simulink model "ER16_Simulation_Line_2020a"  (R2020a)
settings: Solver=ode15s  StartTime=0.0  StopTime=50  RelTol=1e-3
PreLoadFcn:
  | run('ER16_DataFile.m'); % 手动加载模型装配数据
model workspace: external: MATLAB File E:\Traj-tracking Simulation of ER16\Code\ER16_DataFile.m (data not in the file)
undefined symbols (not defined in the file): sigbuilder_block, smiData, X, Y, Z
libraries: sm_lib x49, nesl_utility x13
(part 2 of 2)

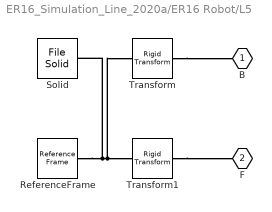
== system ER16_Simulation_Line_2020a/ER16 Robot/L5 ==
  ReferenceFrame : sm_lib/Frames and Transforms/Reference Frame
  Solid : sm_lib/Body Elements/File Solid  ExtGeomFileName=..\3D-Models\ER16_j5_默认_sldprt.STL  UnitType=Custom  ExtGeomFileUnits=mm  StepReaderType=HEX  ExportConvexHullGeometry=off  InertiaType=Custom  Mass=smiData.Solid(5).mass  MassUnits=kg  CenterOfMass=smiData.Solid(5).CoM  CenterOfMassUnits=mm  MomentsOfInertia=smiData.Solid(5).MoI  MomentsOfInertiaUnits=kg*mm^2  ProductsOfInertia=smiData.Solid(5).PoI  ProductsOfInertiaUnits=kg*mm^2  BasedOnType=DensityFromFile  Density=1000  DensityUnits=kg/m^3  DoExposeReferenceFrame=on  SerializedFrames=<Frames/>  GraphicType=FromGeometry  MarkerShape=Sphere  MarkerSize=10  GraphicVisPropType=SimpleVisualProperties  GraphicDiffuseColor=[0.82 0.49 0.11]  GraphicSpecularColor=[0.5 0.5 0.5 1.0]  GraphicAmbientColor=[0.15 0.15 0.15 1.0]  GraphicEmissiveColor=[0.0 0.0 0.0 1.0]  GraphicShininess=75  GraphicOpacity=smiData.Solid(5).opacity
  Transform : sm_lib/Frames and Transforms/Rigid Transform  TranslationMethod=Cartesian  TranslationStandardOffset=0  TranslationLengthUnit=mm  TranslationStandardAxis=+Z  TranslationCartesianOffset=smiData.RigidTransform(12).translation  TranslationROffset=0  TranslationROffsetUnits=m  TranslationZOffset=0  TranslationZOffsetUnits=m  TranslationThetaOffset=0  TranslationThetaOffsetUnits=deg  RotationMethod=ArbitraryAxis  RotationAngleUnits=rad  RotationStandardAxis=+Z  RotationAngle=smiData.RigidTransform(12).angle  RotationArbitraryAxis=smiData.RigidTransform(12).axis  FollAlignAxisA=+X  BaseAlignAxisA=+Y  FollAlignAxisB=+Y  BaseAlignAxisB=+Z  RotationSequenceAxes=FollowerAxes  RotationSequence=XYX  RotationSequenceAngles=[0 0 0]  RotationSequenceAnglesUnits=deg  RotationMatrix=[1 0 0; 0 1 0; 0 0 1]
  Transform1 : sm_lib/Frames and Transforms/Rigid Transform  TranslationMethod=Cartesian  TranslationStandardOffset=0  TranslationLengthUnit=mm  TranslationStandardAxis=+Z  TranslationCartesianOffset=smiData.RigidTransform(13).translation  TranslationROffset=0  TranslationROffsetUnits=m  TranslationZOffset=0  TranslationZOffsetUnits=m  TranslationThetaOffset=0  TranslationThetaOffsetUnits=deg  RotationMethod=ArbitraryAxis  RotationAngleUnits=rad  RotationStandardAxis=+Z  RotationAngle=smiData.RigidTransform(13).angle  RotationArbitraryAxis=smiData.RigidTransform(13).axis  FollAlignAxisA=+X  BaseAlignAxisA=+Y  FollAlignAxisB=+Y  BaseAlignAxisB=+Z  RotationSequenceAxes=FollowerAxes  RotationSequence=XYX  RotationSequenceAngles=[0 0 0]  RotationSequenceAnglesUnits=deg  RotationMatrix=[1 0 0; 0 1 0; 0 0 1]
  B : PMIOPort  Side=Left
  F : PMIOPort  Port=2  Side=Right
  connections:
  Solid/RConn1 -- ReferenceFrame/RConn1 -- Transform/LConn1 -- Transform1/LConn1
  Transform/RConn1 -- B/RConn1
  Transform1/RConn1 -- F/RConn1

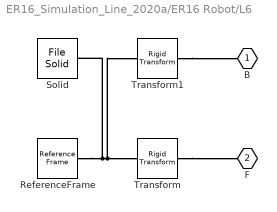
== system ER16_Simulation_Line_2020a/ER16 Robot/L6 ==
  ReferenceFrame : sm_lib/Frames and Transforms/Reference Frame
  Solid : sm_lib/Body Elements/File Solid  ExtGeomFileName=..\3D-Models\ER16_j6_默认_sldprt.STL  UnitType=Custom  ExtGeomFileUnits=mm  StepReaderType=HEX  ExportConvexHullGeometry=off  InertiaType=Custom  Mass=smiData.Solid(1).mass  MassUnits=kg  CenterOfMass=smiData.Solid(1).CoM  CenterOfMassUnits=mm  MomentsOfInertia=smiData.Solid(1).MoI  MomentsOfInertiaUnits=kg*mm^2  ProductsOfInertia=smiData.Solid(1).PoI  ProductsOfInertiaUnits=kg*mm^2  BasedOnType=DensityFromFile  Density=1000  DensityUnits=kg/m^3  DoExposeReferenceFrame=on  SerializedFrames=<Frames/>  GraphicType=FromGeometry  MarkerShape=Sphere  MarkerSize=10  GraphicVisPropType=SimpleVisualProperties  GraphicDiffuseColor=[0.82 0.49 0.11]  GraphicSpecularColor=[0.5 0.5 0.5 1.0]  GraphicAmbientColor=[0.15 0.15 0.15 1.0]  GraphicEmissiveColor=[0.0 0.0 0.0 1.0]  GraphicShininess=75  GraphicOpacity=smiData.Solid(1).opacity
  Transform : sm_lib/Frames and Transforms/Rigid Transform  TranslationMethod=Cartesian  TranslationStandardOffset=0  TranslationLengthUnit=mm  TranslationStandardAxis=+Z  TranslationCartesianOffset=smiData.RigidTransform(1).translation  TranslationROffset=0  TranslationROffsetUnits=m  TranslationZOffset=0  TranslationZOffsetUnits=m  TranslationThetaOffset=0  TranslationThetaOffsetUnits=deg  RotationMethod=ArbitraryAxis  RotationAngleUnits=rad  RotationStandardAxis=+Z  RotationAngle=smiData.RigidTransform(1).angle  RotationArbitraryAxis=smiData.RigidTransform(1).axis  FollAlignAxisA=+X  BaseAlignAxisA=+Y  FollAlignAxisB=+Y  BaseAlignAxisB=+Z  RotationSequenceAxes=FollowerAxes  RotationSequence=XYX  RotationSequenceAngles=[0 0 0]  RotationSequenceAnglesUnits=deg  RotationMatrix=[1 0 0; 0 1 0; 0 0 1]
  Transform1 : sm_lib/Frames and Transforms/Rigid Transform  TranslationMethod=Cartesian  TranslationStandardOffset=0  TranslationLengthUnit=mm  TranslationStandardAxis=+Z  TranslationCartesianOffset=smiData.RigidTransform(14).translation  TranslationROffset=0  TranslationROffsetUnits=m  TranslationZOffset=0  TranslationZOffsetUnits=m  TranslationThetaOffset=0  TranslationThetaOffsetUnits=deg  RotationMethod=ArbitraryAxis  RotationAngleUnits=rad  RotationStandardAxis=+Z  RotationAngle=smiData.RigidTransform(14).angle  RotationArbitraryAxis=smiData.RigidTransform(14).axis  FollAlignAxisA=+X  BaseAlignAxisA=+Y  FollAlignAxisB=+Y  BaseAlignAxisB=+Z  RotationSequenceAxes=FollowerAxes  RotationSequence=XYX  RotationSequenceAngles=[0 0 0]  RotationSequenceAnglesUnits=deg  RotationMatrix=[1 0 0; 0 1 0; 0 0 1]
  B : PMIOPort  Side=Left
  F : PMIOPort  Port=2  Side=Right
  connections:
  Solid/RConn1 -- ReferenceFrame/RConn1 -- Transform/LConn1 -- Transform1/LConn1
  Transform/RConn1 -- F/RConn1
  Transform1/RConn1 -- B/RConn1

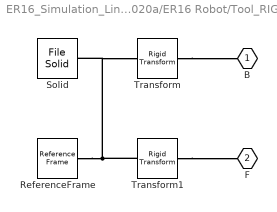
== system ER16_Simulation_Line_2020a/ER16 Robot/Tool_RIGID ==
  ReferenceFrame : sm_lib/Frames and Transforms/Reference Frame
  Solid : sm_lib/Body Elements/File Solid  ExtGeomFileName=..\3D-Models\Tool_默认_sldprt.STL  UnitType=Custom  ExtGeomFileUnits=mm  StepReaderType=HEX  ExportConvexHullGeometry=off  InertiaType=Custom  Mass=smiData.Solid(9).mass  MassUnits=kg  CenterOfMass=smiData.Solid(9).CoM  CenterOfMassUnits=mm  MomentsOfInertia=smiData.Solid(9).MoI  MomentsOfInertiaUnits=kg*mm^2  ProductsOfInertia=smiData.Solid(9).PoI  ProductsOfInertiaUnits=kg*mm^2  BasedOnType=DensityFromFile  Density=1000  DensityUnits=kg/m^3  DoExposeReferenceFrame=on  SerializedFrames=<Frames/>  GraphicType=FromGeometry  MarkerShape=Sphere  MarkerSize=10  GraphicVisPropType=SimpleVisualProperties  GraphicDiffuseColor=smiData.Solid(9).color  GraphicSpecularColor=[0.5 0.5 0.5 1.0]  GraphicAmbientColor=[0.15 0.15 0.15 1.0]  GraphicEmissiveColor=[0.0 0.0 0.0 1.0]  GraphicShininess=75  GraphicOpacity=smiData.Solid(9).opacity
  Transform : sm_lib/Frames and Transforms/Rigid Transform  TranslationMethod=Cartesian  TranslationStandardOffset=0  TranslationLengthUnit=mm  TranslationStandardAxis=+Z  TranslationCartesianOffset=smiData.RigidTransform(2).translation  TranslationROffset=0  TranslationROffsetUnits=m  TranslationZOffset=0  TranslationZOffsetUnits=m  TranslationThetaOffset=0  TranslationThetaOffsetUnits=deg  RotationMethod=ArbitraryAxis  RotationAngleUnits=rad  RotationStandardAxis=+Z  RotationAngle=smiData.RigidTransform(2).angle  RotationArbitraryAxis=smiData.RigidTransform(2).axis  FollAlignAxisA=+X  BaseAlignAxisA=+Y  FollAlignAxisB=+Y  BaseAlignAxisB=+Z  RotationSequenceAxes=FollowerAxes  RotationSequence=XYX  RotationSequenceAngles=[0 0 0]  RotationSequenceAnglesUnits=deg  RotationMatrix=[1 0 0; 0 1 0; 0 0 1]
  Transform1 : sm_lib/Frames and Transforms/Rigid Transform  TranslationMethod=Cartesian  TranslationStandardOffset=0.1325  TranslationLengthUnit=mm  TranslationStandardAxis=+X  TranslationCartesianOffset=smiData.RigidTransform(2).translation  TranslationROffset=0  TranslationROffsetUnits=m  TranslationZOffset=0  TranslationZOffsetUnits=m  TranslationThetaOffset=0  TranslationThetaOffsetUnits=deg  RotationMethod=ArbitraryAxis  RotationAngleUnits=rad  RotationStandardAxis=+Z  RotationAngle=0  RotationArbitraryAxis=smiData.RigidTransform(2).axis  FollAlignAxisA=+X  BaseAlignAxisA=+Y  FollAlignAxisB=+Y  BaseAlignAxisB=+Z  RotationSequenceAxes=FollowerAxes  RotationSequence=XYX  RotationSequenceAngles=[0 0 0]  RotationSequenceAnglesUnits=deg  RotationMatrix=[1 0 0; 0 1 0; 0 0 1]
  B : PMIOPort  Side=Left
  F : PMIOPort  Port=2  Side=Right
  connections:
  ReferenceFrame/RConn1 -- Transform1/LConn1 -- Transform/LConn1 -- Solid/RConn1
  Transform/RConn1 -- B/RConn1
  Transform1/RConn1 -- F/RConn1

== matlab function ER16_Simulation_Line_2020a/Calculator/Impedance Control Y ==
  settings: updateMethod=DISCRETE  sampleTime=0.005
  data: Y_Xd input; Y_Xr output; Y_Xr_d output; Y_Xr_dd output; Y_Xd_d input; Y_Xd_dd input; f input
function [Y_Xr,Y_Xr_d,Y_Xr_dd]  = fcnlmp(Y_Xd,Y_Xd_d,Y_Xd_dd,f)
m =1;b = 200;k=300;T = 0.005; % 参数初始化
persistent Xr_pre Xr_dot_pre;% 持久变量 https://ww2.mathworks.cn/help/matlab/ref/persistent.html
if isempty(Xr_pre) 
    Xr_pre = 0;
end
if isempty(Xr_dot_pre) 
    Xr_dot_pre = 0;
end
Xr_dotdot_pre = Y_Xd_dd + 1/m*(-f + b*(Y_Xd_d - Xr_dot_pre) + k*(Y_Xd - Xr_pre)); % 上一采样时间 nT 机器人末端的实际运动加速度
Y_Xr = Xr_pre + Xr_dot_pre*T;         % 当前采样时间 (n+1)T 机器人末端的实际运动位置
Y_Xr_d = Xr_dot_pre + Xr_dotdot_pre*T;% 当前采样时间 (n+1)T 机器人末端的实际运动速度
Y_Xr_dd = Xr_dotdot_pre;              % 当前采样时间 (n+1)T 机器人末端的实际运动加速度
Xr_dot_pre = Y_Xr_d;                  % 上一采样时间 nT 机器人末端的实际运动速度
Xr_pre = Y_Xr;                        % 上一采样时间 nT 机器人末端的实际运动位置
end

== matlab function ER16_Simulation_Line_2020a/Calculator/Impedance Control X ==
  settings: updateMethod=DISCRETE  sampleTime=0.005
  data: X_Xd input; X_Xr output; X_Xr_d output; X_Xr_dd output; X_Xd_d input; X_Xd_dd input; f input
function [X_Xr,X_Xr_d,X_Xr_dd]  = fcnlmp(X_Xd,X_Xd_d,X_Xd_dd,f)
m =1;b = 200;k= 300;T = 0.005; % 参数初始化
persistent Xr_pre Xr_dot_pre;% 持久变量 https://ww2.mathworks.cn/help/matlab/ref/persistent.html
if isempty(Xr_pre) 
    Xr_pre = 0;
end
if isempty(Xr_dot_pre) 
    Xr_dot_pre = 0;
end
Xr_dotdot_pre = X_Xd_dd + 1/m*(-f + b*(X_Xd_d - Xr_dot_pre) + k*(X_Xd - Xr_pre)); % 上一采样时间 nT 机器人末端的实际运动加速度
X_Xr = Xr_pre + Xr_dot_pre*T;         % 当前采样时间 (n+1)T 机器人末端的实际运动位置
X_Xr_d = Xr_dot_pre + Xr_dotdot_pre*T;% 当前采样时间 (n+1)T 机器人末端的实际运动速度
X_Xr_dd = Xr_dotdot_pre;              % 当前采样时间 (n+1)T 机器人末端的实际运动加速度
Xr_dot_pre = X_Xr_d;                  % 上一采样时间 nT 机器人末端的实际运动速度
Xr_pre = X_Xr;                        % 上一采样时间 nT 机器人末端的实际运动位置
end

== matlab function ER16_Simulation_Line_2020a/Calculator/Impedance Control Z ==
  settings: updateMethod=DISCRETE  sampleTime=0.005
  data: Z_Xd input; Z_Xr output; Z_Xr_d output; Z_Xr_dd output; Z_Xd_d input; Z_Xd_dd input; f input
function [Z_Xr,Z_Xr_d,Z_Xr_dd]  = fcnlmp(Z_Xd,Z_Xd_d,Z_Xd_dd,f)
m =1;b = 200;k=300;T = 0.005; % 参数初始化
persistent Xr_pre Xr_dot_pre;% 持久变量 https://ww2.mathworks.cn/help/matlab/ref/persistent.html
if isempty(Xr_pre) 
    Xr_pre = 0;
end
if isempty(Xr_dot_pre) 
    Xr_dot_pre = 0;
end
Xr_dotdot_pre = Z_Xd_dd + 1/m*(-f + b*(Z_Xd_d - Xr_dot_pre) + k*(Z_Xd - Xr_pre)); % 上一采样时间 nT 机器人末端的实际运动加速度
Z_Xr = Xr_pre + Xr_dot_pre*T;           % 当前采样时间 (n+1)T 机器人末端的实际运动位置
Z_Xr_d = Xr_dot_pre + Xr_dotdot_pre*T;% 当前采样时间 (n+1)T 机器人末端的实际运动速度
Z_Xr_dd = Xr_dotdot_pre;            % 当前采样时间 (n+1)T 机器人末端的实际运动加速度
Xr_dot_pre = Z_Xr_d;                  % 上一采样时间 nT 机器人末端的实际运动速度
Xr_pre = Z_Xr;                          % 上一采样时间 nT 机器人末端的实际运动位置
end

== matlab function ER16_Simulation_Line_2020a/Trajectory Planner /Trajectory ==
  data: Mode input; Traj output; Clock input; Stoptime input
function Traj = traj(Mode,Clock,Stoptime)
    if Mode == 0 % 圆周轨迹
        theta = 2*pi*Clock/Stoptime;
        Xd = 0.2*cos(theta)-0.2;
        Yd = 0;
        Zd = 0.2*sin(theta);
        Traj = [Xd;Yd;Zd];
    else        % 直线轨迹
        Xd = 0;
        Yd = 0;
        Zd = 0.2*Clock/Stoptime;
        Traj = [Xd;Yd;Zd];
    end
end
